simulink subsystem "Parachute_model"  (R2024b)
settings: Solver=VariableStepAuto  StartTime=0.0  StopTime=10.0  RelTol=1e-3
model mask{radius=0, Cd=0, parachute_deployment_type=ParachuteDeploymentType.Apogee_Delay_Deployment, burnout_delay=0, deploy_height=0}
  mask prompts: radius "Parachute Radius"; Cd "Parachute Drag Coefficient"; parachute_deployment_type "Parachute Deployment Type"; burnout_delay "Parachute Burnout Delay"; deploy_height "Parachute Deployment Height"
values from neighbouring files (symbols this model uses):
  deploy_height = 0    [Parachute.m]
undefined symbols (not defined in the file or in its folder): XCG_dry
settings Model: Creator=thatf  LastModifiedBy=thatf
settings RTWCC: GPUComputeCapability=3.5

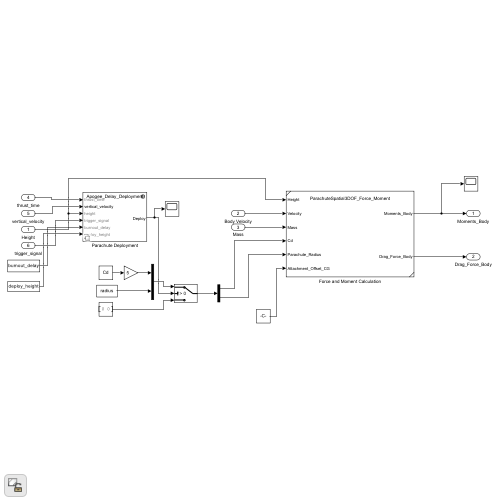
[thumbnail: Simulink's stored preview of the top-level diagram]
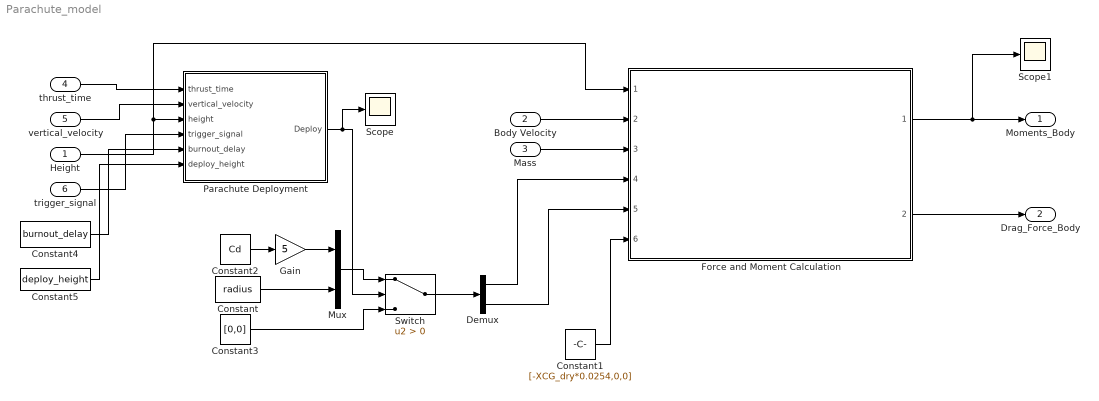
== system Parachute_model ==
  Height : Inport
  Body Velocity : Inport  Port=2
  Mass : Inport  Port=3
  thrust_time : Inport  Port=4
  vertical_velocity : Inport  Port=5
  trigger_signal : Inport  Port=6
  Constant : Constant  Value=radius
  Constant1 : Constant  Value=[-XCG_dry*0.0254,0,0]
  Constant2 : Constant  Value=Cd
  Constant3 : Constant  Value=[0,0]
  Constant4 : Constant  Value=burnout_delay
  Constant5 : Constant  Value=deploy_height
  Demux : Demux  Outputs=2
  Force and Moment Calculation : Subsystem  ReferencedSubsystem=ParachuteSpatial3DOF_Force_Moment
  Gain : Gain  Gain=5
  Mux : Mux  Inputs=2
  Parachute Deployment : Subsystem  Variant=on  VariantChoicesSpecifier={'Parachute_Deployment_Systems/*.slx'}  VariantChoicesEnumeration=ParachuteDeploymentType  VariantControlVariable=parachute_deployment_type
  Scope : Scope
  Scope1 : Scope
  Switch : Switch  Criteria=u2 > Threshold  SaturateOnIntegerOverflow=off  InputSameDT=off
  Moments_Body : Outport
  Drag_Force_Body : Outport  Port=2
  wires:
  Constant1/1 -> Force and Moment Calculation/6
  Body Velocity/1 -> Force and Moment Calculation/2
  Mass/1 -> Force and Moment Calculation/3
  Parachute Deployment/1(Deploy) -> Switch/2, Scope/1
  Constant3/1 -> Switch/3
  Force and Moment Calculation/1 -> Moments_Body/1, Scope1/1
  Force and Moment Calculation/2 -> Drag_Force_Body/1
  Height/1 -> Force and Moment Calculation/1, Parachute Deployment/3(height)
  thrust_time/1 -> Parachute Deployment/1(thrust_time)
  vertical_velocity/1 -> Parachute Deployment/2(vertical_velocity)
  Switch/1 -> Demux/1
  Demux/1 -> Force and Moment Calculation/4
  Demux/2 -> Force and Moment Calculation/5
  Mux/1 -> Switch/1
  Constant/1 -> Mux/2
  trigger_signal/1 -> Parachute Deployment/4(trigger_signal)
  Constant4/1 -> Parachute Deployment/5(burnout_delay)
  Constant5/1 -> Parachute Deployment/6(deploy_height)
  Constant2/1 -> Gain/1
  Gain/1 -> Mux/1

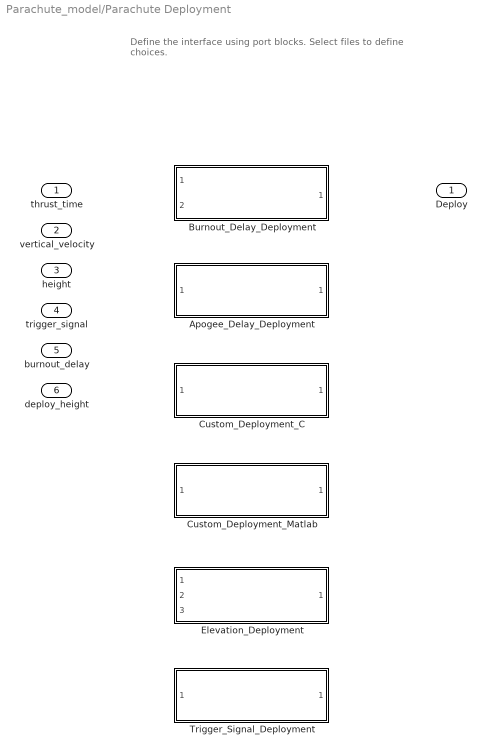
== system Parachute_model/Parachute Deployment ==
  note: Define the interface using port blocks.
      | Select files to define choices.
  thrust_time : Inport
  vertical_velocity : Inport  Port=2
  height : Inport  Port=3
  trigger_signal : Inport  Port=4
  burnout_delay : Inport  Port=5
  deploy_height : Inport  Port=6
  Apogee_Delay_Deployment : Subsystem  VariantControl=parachute_deployment_type == ParachuteDeploymentType.Apogee_Delay_Deployment  ReferencedSubsystem=Apogee_Delay_Deployment
  Burnout_Delay_Deployment : Subsystem  VariantControl=parachute_deployment_type == ParachuteDeploymentType.Burnout_Delay_Deployment  ReferencedSubsystem=Burnout_Delay_Deployment
  Custom_Deployment_C : Subsystem  VariantControl=parachute_deployment_type == ParachuteDeploymentType.Custom_Deployment_C  ReferencedSubsystem=Custom_Deployment_C
  Custom_Deployment_Matlab : Subsystem  VariantControl=parachute_deployment_type == ParachuteDeploymentType.Custom_Deployment_Matlab  ReferencedSubsystem=Custom_Deployment_Matlab
  Elevation_Deployment : Subsystem  VariantControl=parachute_deployment_type == ParachuteDeploymentType.Elevation_Deployment  ReferencedSubsystem=Elevation_Deployment
  Trigger_Signal_Deployment : Subsystem  VariantControl=parachute_deployment_type == ParachuteDeploymentType.Trigger_Signal_Deployment  ReferencedSubsystem=Trigger_Signal_Deployment
  Deploy : Outport
